simulink model "Ship"  (Simulink 8.3)
settings: Solver=ode45  StartTime=0.0  StopTime=10.0  RelTol=1e-3
undefined symbols (not defined in the file): k, m
settings Model: Creator=Administrator  LastModifiedBy=Administrator
settings DataIOCC: SignalLoggingSaveFormat=Dataset
settings DebuggingCC: UnderspecifiedInitializationDetection=Simplified  StateNameClashWarn=none
settings GRTTargetCC: CombineOutputUpdateFcns=on  GRTInterface=off

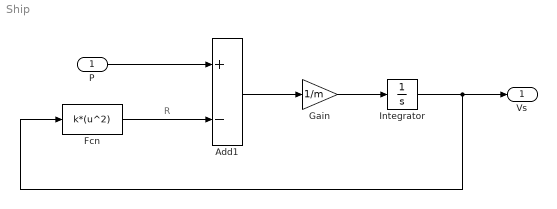
== system Ship ==
  note: R
  P : Inport
  Add1 : Sum  Inputs=+-
  Fcn : Fcn  Expr=k*(u^2)
  Gain : Gain  Gain=1/m
  Integrator : Integrator
  Vs : Outport
  wires:
  P/1 -> Add1/1
  Fcn/1 -> Add1/2
  Add1/1 -> Gain/1
  Gain/1 -> Integrator/1
  Integrator/1 -> Vs/1, Fcn/1
